simulink subsystem "NoTrailer"  (R2024b)
settings: Solver=VariableStepAuto  StartTime=0.0  StopTime=10.0  RelTol=1e-3
settings Model: ModifiedByFormat=The MathWorks, Inc.  Creator=The MathWorks, Inc.  LastModifiedBy=The MathWorks, Inc.
settings RTWCC: GPUComputeCapability=3.5

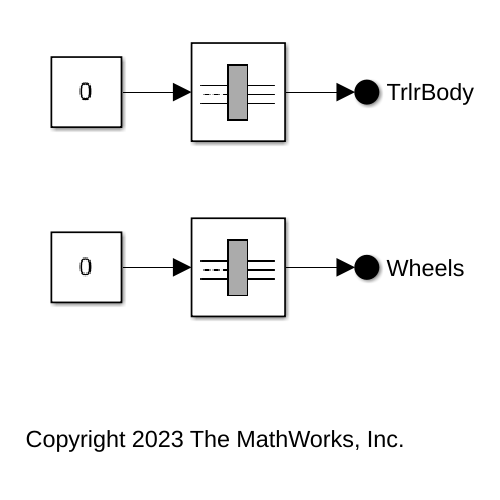
[thumbnail: Simulink's stored preview of the top-level diagram]
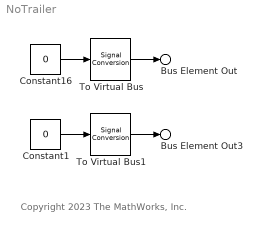
== system NoTrailer ==
  note: Copyright 2023 The MathWorks, Inc.
  Constant1 : Constant  Value=0  OutDataTypeStr=Bus: TrlrWheelsBUS  SampleTime=Inf
  Constant16 : Constant  Value=0  OutDataTypeStr=Bus: TrlrBodyBUS  SampleTime=Inf
  To Virtual Bus : SignalConversion  ConversionOutput=Virtual bus  OverrideOpt=off
  To Virtual Bus1 : SignalConversion  ConversionOutput=Virtual bus  OverrideOpt=off
  Bus Element Out3 : Outport  PortName=Wheels
  Bus Element Out : Outport  Port=2  PortName=TrlrBody
  wires:
  To Virtual Bus1/1 -> Bus Element Out3/1
  To Virtual Bus/1 -> Bus Element Out/1
  Constant1/1 -> To Virtual Bus1/1
  Constant16/1 -> To Virtual Bus/1
